simulink model "CarLike_Robot"  (R2024b)
settings: Solver=FixedStepAuto  StartTime=0.0  StopTime=T_max  FixedStep=Ts  RelTol=1e-3
StopFcn:
  | %plot_trajectory(out.x.Data(:,1), out.y.Data(:,1), 'x [m]', 'y [m]', fullfile('C:\Users\paolo\OneDrive - MSFT\Documenti\Personali\Scuola\università\magistrale\2° ANNO\Secondo Semestre\FSR\Project\Software\Images\Paper\Chapter_4_simulation\RSC\simulink', 'current_trajectory.pdf'));
  | %plot_trajectory(out.x_d.Data(1,:), out.y_d.Data(1,:), '$x_d$ [m]', '$y_d$ [m]', fullfile('C:\Users\paolo\OneDrive - MSFT\Documenti\Personali\Scuola\università\magistrale\2° ANNO\Secondo Semestre\FSR\Project\Software\Images\Paper\Chapter_4_simulation\RSC\simulink', 'desidered_trajectory.pdf'));
  | %plot_velocity(out.v.Time, out.omega.Time, out.v.Data(:,1), out.omega.Data(:,1), 'time [s]', 'v [m/s]', '$\omega$ [rad/s]', fullfile('C:\Users\paolo\OneDrive - MSFT\Documenti\Personali\Scuola\università\magistrale\2° ANNO\Secondo Semestre\FSR\Project\Software\Images\Paper\Chapter_4_simulation\RSC\simulink', 'velocity.pdf'));
  | %plot_error(out.x.Time, out.x_d.Data(1,:), out.x.Data(:,1), 'time [s]', '$e_x$ [m]', fullfile('C:\Users\paolo\OneDrive - MSFT\Documenti\Personali\Scuola\università\magistrale\2° ANNO\Secondo Semestre\FSR\Project\Software\Images\Paper\Chapter_4_simulation\RSC\simulink', 'error_x.pdf'));
  | %plot_error(out.y.Time, out.y_d.Data(1,:), out.y.Data(:,1), 'time [s]', '$e_y$ [m]', fullfile('C:\Users\paolo\OneDrive - MSFT\Documenti\Personali\Scuola\università\magistrale\2° ANNO\Secondo Semestre\FSR\Project\Software\Images\Paper\Chapter_4_simulation\RSC\simulink', 'error_y.pdf'));
  | %plot_error(out.theta.Time, out.theta_d.Data(1,:), out.theta.Data(:,1), 'time [s]', '$e_{\theta}$ [rad]', fullfile('C:\Users\paolo\OneDrive - MSFT\Documenti\Personali\Scuola\università\magistrale\2° ANNO\Secondo Semestre\FSR\Project\Software\Images\Paper\Chapter_4_simulation\RSC\simulink', 'error_theta.pdf'));
  | %plot_error(out.phi.Time, out.phi_d.Data(1,:), out.phi.Data(:,1), 'time [s]', '$e_{\phi}$ [rad]', fullfile('C:\Users\paolo\OneDrive - MSFT\Documenti\Personali\Scuola\università\magistrale\2° ANNO\Secondo Semestre\FSR\Project\Software\Images\Paper\Chapter_4_simulation\RSC\simulink', 'error_phi.pdf'));
values from neighbouring files (symbols this model uses):
  Delta = 0.2    [main.m]
  l = 0.6    [main.m]
  landmarks = zeros(num_landmarks, 2)    [main.m]
  localization = choice - 1    [main.m]
  omega_max_ref = max(abs(omega))    [main.m]
  P0 = eye(4) * 0.1    [main.m]
  q0 = [xd0; yd0; thetad0; phid0]    [main.m]
  Q_ekf = diag([0.01, 0.01])    [main.m]
  R_ekf = diag([0.05, 0.02])    [main.m]
  Ts = 0.01    [main.m]
  v_max_ref = max(abs(v))    [main.m]
  y_1d_goal = xd_end + l*cos(thetad_end) + Delta*cos(thetad_end + phid_end)    [main.m]
  y_2d_goal = yd_end + l*sin(thetad_end) + Delta*sin(thetad_end + phid_end)    [main.m]
libraries: robotmobilelib x1
settings Model: LastModifiedBy=lowan
settings SolverCC: EnableFixedStepZeroCrossing=on
settings ModelReferenceCC: EnableRefExpFcnMdlSchedulingChecks=on
settings RTWCC: GPUComputeCapability=3.5

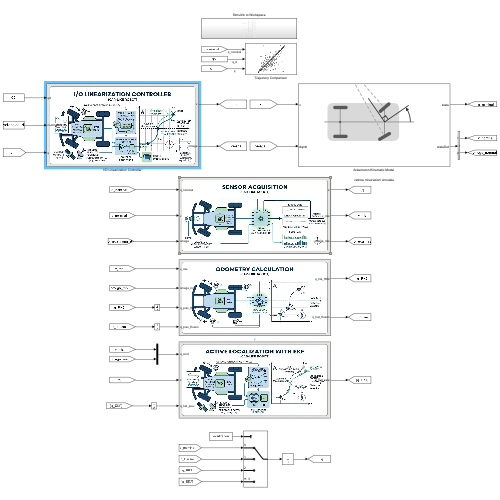
[thumbnail: Simulink's stored preview of the top-level diagram]
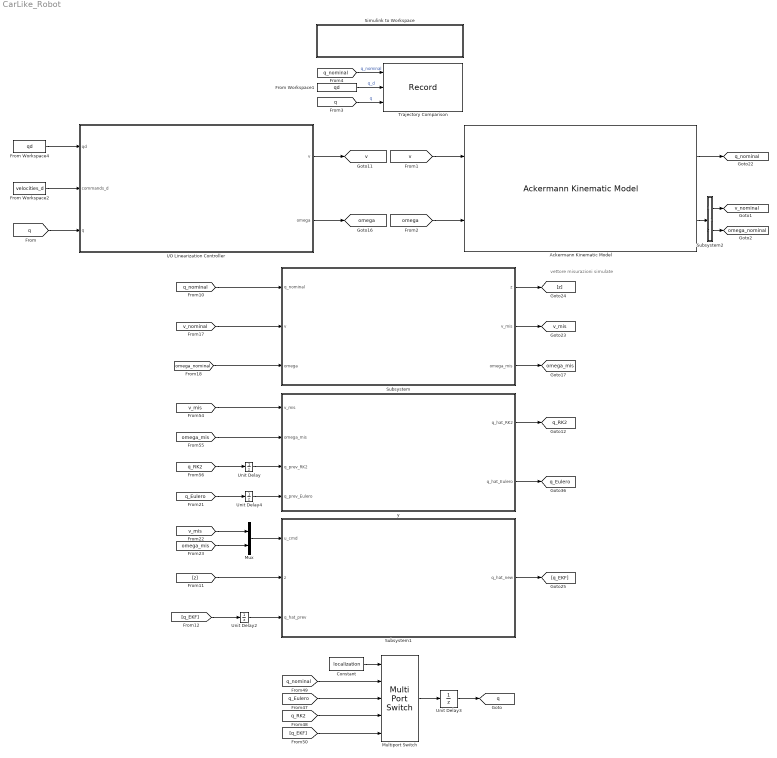
== system CarLike_Robot ==
  note: vettore misurazioni simulate
  "Ackermann Kinematic Model " : robotmobilelib/Ackermann Kinematic Model  WheelBase=0.6  VehicleSpeedRange=[-3 3]  MaxSteeringAngle=pi/4  InitialState=q0  SimulateUsing=Interpreted execution
  Constant : Constant  Value=localization
  From Workspace1 : FromWorkspace  VariableName=qd  SampleTime=Ts  OutputAfterFinalValue=Holding final value
  From Workspace2 : FromWorkspace  VariableName=velocities_d  SampleTime=Ts  OutputAfterFinalValue=Holding final value
  From Workspace4 : FromWorkspace  VariableName=qd  SampleTime=Ts  OutputAfterFinalValue=Holding final value
  I/O Linearization Controller : Subsystem
      mask Display: image('IO_Linearization_Controller.png');
  Multiport Switch : MultiPortSwitch  DataPortOrder=Zero-based contiguous  Inputs=4  zeroidx=on  SaturateOnIntegerOverflow=off  InputSameDT=off
  Mux : Mux  Inputs=2
  Simulink to Workspace : Subsystem
  Subsystem : Subsystem
      mask Display: image('Sensors.png');
  Subsystem1 : Subsystem
      mask Display: image('Active_Localization_EKF.png');
  Subsystem2 : Subsystem
  Trajectory Comparison : Record  FileSettingsInternal="{\"entries\":[{\"content\":{\"excelSettings\":{\"content\":{},\"type\":\"Streamout.ExcelSettings\"}},\"type\":\"Streamout.FileSettingStorage\",\"uuid\":\"\"}],\"packageUris\":[\"http:\\/\\/schema.mathworks.com\\/mf0\\/streamout_blocks\\/R2020a\"],\"version\":\"1.0\"}"  Layout=[1 1]  SignalsInternal="{\"entries\":[{\"content\":{\"signals\":[{\"content\":{\"blockPath\":[],\"dimensions\":[4],\"domain\":\"\",\"hasChildren\":true,\"lineColor\":\"#ff6929\",\"lineWidth\":2,\"port\":1,\"sid\":[\"\"],\"signalID\":1,\"signalName\":\"q_nominal\"},\"type\":\"RecordBlkView.Signal\",\"uuid\":\"\"},{\"content\":{\"blockPath\":[],\"channel\":[1],\"dimensions\":[4],\"domain\":\"\",\"lineColor\":\"#139fff\",\"lineWidth\":2,\"parentID\":1,\"plots\":[ 1 ],\"port\":1,\"sid\":[\"\"],\"signalID\":2,\"signalName\":\"q_nominal\"},\"type\":\"RecordBlkView.Signal\",\"uuid\":\"\"},{\"content\":{\"blockPath\":[],\"dimensions\":[4],\"domain\":\"\",\"hasChildren\":true,\"lineColor\":\"#64d413\",\"lineWidth\":2,\"port\":2,\"sid\":[\"\"],\"signalID\":3,\"signalName\":\"q_d\"},\"type\":\"RecordBlkView.Signal\",\"uuid\":\"\"},{\"content\":{\"blockPath\":[],\"channel\":[1],\"dimensions\":[4],\"domain\":\"\",\"lineColor\":\"#b746ff\",\"lineWidth\":2,\"parentID\":3,\"plots\":[ 1 ],\"port\":2,\"sid\":[\"\"],\"signalID\":4,\"signalName\":\"q_d\"},\"type\":\"RecordBlkView.Signal\",\"uuid\":\"\"},{\"content\":{\"blockPath\":[],\"dimensions\":[4,1],\"domain\":\"\",\"hasChildren\":true,\"lineColor\":\"#fe330a\",\"lineWidth\":2,\"port\":3,\"sid\":[\"\"],\"signalID\":5,\"signalName\":\"q\"},\"type\":\"RecordBlkView.Signal\",\"uuid\":\"\"},{\"content\":{\"blockPath\":[],\"channel\":[1,1],\"dimensions\":[4,1],\"domain\":\"\",\"lineColor\":\"#4dbeee\",\"lineWidth\":2,\"parentID\":5,\"plots\":[ 1 ],\"port\":3,\"sid\":[\"\"],\"signalID\":6,\"signalName\":\"q\"},\"type\":\"RecordBlkView.Signal\",\"uuid\":\"\"},{\"content\":{\"blockPath\":[],\"channel\":[2],\"dimensions\":[4],\"domain\":\"\",\"lineColor\":\"#a2142f\",\"lineWidth\":2,\"parentID\":1,\"plots\":[ 1 ],\"port\":1,\"sid\":[\"\"],\"signalID\":7,\"signalName\":\"q_nominal\"},\"type\":\"RecordBlkView.Signal\",\"uuid\":\"\"},{\"content\":{\"blockPath\":[],\"channel\":[3],\"dimensions\":[4],\"domain\":\"\",\"lineColor\":\"#139fff\",\"lineWidth\":2,\"parentID\":1,\"port\":1,\"sid\":[\"\"],\"signalID\":8,\"signalName\":\"q_nominal\"},\"type\":\"RecordBlkView.Signal\",\"uuid\":\"\"},{\"content\":{\"blockPath\":[],\"channel\":[4],\"dimensions\":[4],\"domain\":\"\",\"lineColor\":\"#ff6929\",\"lineWidth\":2,\"parentID\":1,\"port\":1,\"sid\":[\"\"],\"signalID\":9,\"signalName\":\"q_nominal\"},\"type\":\"RecordBlkView.Signal\",\"uuid\":\"\"},{\"content\":{\"blockPath\":[],\"channel\":[2],\"dimensions\":[4],\"domain\":\"\",\"lineColor\":\"#b746ff\",\"lineWidth\":2,\"parentID\":3,\"plots\":[ 1 ],\"port\":2,\"sid\":[\"\"],\"signalID\":10,\"signalName\":\"q_d\"},\"type\":\"RecordBlkView.Signal\",\"uuid\":\"\"},{\"content\":{\"blockPath\":[],\"channel\":[3],\"dimensions\":[4],\"domain\":\"\",\"lineColor\":\"#64d413\",\"lineWidth\":2,\"parentID\":3,\"port\":2,\"sid\":[\"\"],\"signalID\":11,\"signalName\":\"q_d\"},\"type\":\"RecordBlkView.Signal\",\"uuid\":\"\"},{\"content\":{\"blockPath\":[],\"channel\":[4],\"dimensions\":[4],\"domain\":\"\",\"lineColor\":\"#ff13a6\",\"lineWidth\":2,\"parentID\":3,\"port\":2,\"sid\":[\"\"],\"signalID\":12,\"signalName\":\"q_d\"},\"type\":\"RecordBlkView.Signal\",\"uuid\":\"\"},{\"content\":{\"blockPath\":[],\"channel\":[2,1],\"dimensions\":[4,1],\"domain\":\"\",\"lineColor\":\"#ff6929\",\"lineWidth\":2,\"parentID\":5,\"plots\":[ 1 ],\"port\":3,\"sid\":[\"\"],\"signalID\":13,\"signalName\":\"q\"},\"type\":\"RecordBlkView.Signal\",\"uuid\":\"\"},{\"content\":{\"blockPath\":[],\"channel\":[3,1],\"dimensions\":[4,1],\"domain\":\"\",\"lineColor\":\"#b746ff\",\"lineWidth\":2,\"parentID\":5,\"port\":3,\"sid\":[\"\"],\"signalID\":14,\"signalName\":\"q\"},\"type\":\"RecordBlkView.Signal\",\"uuid\":\"\"},{\"content\":{\"blockPath\":[],\"channel\":[4,1],\"dimensions\":[4,1],\"domain\":\"\",\"lineColor\":\"#64d413\",\"lineWidth\":2,\"parentID\":5,\"port\":3,\"sid\":[\"\"],\"signalID\":15,\"signalName\":\"q\"},\"type\":\"RecordBlkView.Signal\",\"uuid\":\"\"}]},\"type\":\"RecordBlkView.InputSignals\",\"uuid\":\"\"}],\"packageUris\":[\"http:\\/\\/schema.mathworks.com\\/mf0\\/streamout_blocks\\/R2020a\"],\"version\":\"1.0\"}"  VisualizationBindings="{\"xyplotplugin\":{\"info\":[{\"series\":[{\"bindingParametersList\":[{\"parameter\":\"X-Axis\",\"signalID\":2,\"signalName\":\"q_nominal(1)\"},{\"parameter\":\"Y-Axis\",\"signalID\":7,\"signalName\":\"q_nominal(2)\"}],\"seriesID\":0},{\"bindingParametersList\":[{\"parameter\":\"X-Axis\",\"signalID\":6,\"signalName\":\"q(1,1)\"},{\"parameter\":\"Y-Axis\",\"signalID\":13,\"signalName\":\"q(2,1)\"}],\"seriesID\":1},{\"bindingParametersList\":[{\"parameter\":\"X-Axis\",\"signalID\":4,\"signalName\":\"q_d(1)\"},{\"parameter\":\"Y-Axis\",\"signalID\":10,\"signalName\":\"q_d(2)\"}],\"seriesID\":2}],\"subplotID\":1}]}}"  CompatibilityTag=XY
  Unit Delay{,2..4} (4 alike) : UnitDelay  InitialCondition=q0  SampleTime=Ts  HasFrameUpgradeWarning=on
  y : Subsystem
      mask Display: image('Odometry.png');
  tag scope: omega=global, omega_mis=global, omega_nominal=global, q=global, q_Eulero=global, q_RK2=global, q_nominal=global, v=global, v_mis=global, v_nominal=global
  wires:
  "Ackermann Kinematic Model "/1 -> [q_nominal]
  [q_RK2] -> Unit Delay/1
  [q_EKF] -> Unit Delay2/1
  [v_mis] -> Mux/1
  [omega_mis] -> Mux/2
  [q_Eulero] -> Unit Delay4/1
  [v_mis] -> y/1(v_mis)
  [omega_mis] -> y/2(omega_mis)
  Unit Delay/1 -> y/3(q_prev_RK2)
  Unit Delay4/1 -> y/4(q_prev_Eulero)
  y/1(q_hat_RK2) -> [q_RK2]
  y/2(q_hat_Eulero) -> [q_Eulero]
  [q_nominal] -> Subsystem/1(q_nominal)
  [v_nominal] -> Subsystem/2(v)
  [omega_nominal] -> Subsystem/3(omega)
  Subsystem/1(z) -> [z]
  Subsystem/2(v_mis) -> [v_mis]
  Subsystem/3(omega_mis) -> [omega_mis]
  [omega] -> "Ackermann Kinematic Model "/2
  [q_nominal] -> Multiport Switch/2
  [q_Eulero] -> Multiport Switch/3
  [q_RK2] -> Multiport Switch/4
  [q_EKF] -> Multiport Switch/5
  Constant/1 -> Multiport Switch/1
  Multiport Switch/1 -> Unit Delay3/1
  Unit Delay3/1 -> [q]
  From Workspace4/1 -> I/O Linearization Controller/1(qd)
  [q] -> I/O Linearization Controller/3(q)
  I/O Linearization Controller/1(v) -> [v]
  I/O Linearization Controller/2(omega) -> [omega]
  Mux/1 -> Subsystem1/1(u_cmd)
  [z] -> Subsystem1/2(z)
  Unit Delay2/1 -> Subsystem1/3(q_hat_prev)
  Subsystem1/1(q_hat_new) -> [q_EKF]
  [v] -> "Ackermann Kinematic Model "/1
  From Workspace1/1 -> Trajectory Comparison/2  "q_d"
  [q_nominal] -> Trajectory Comparison/1  "q_nominal"
  From Workspace2/1 -> I/O Linearization Controller/2(commands_d)
  [q] -> Trajectory Comparison/3  "q"
  "Ackermann Kinematic Model "/2 -> Subsystem2/1(In1)
  Subsystem2/1(Out1) -> [v_nominal]
  Subsystem2/2(Out2) -> [omega_nominal]

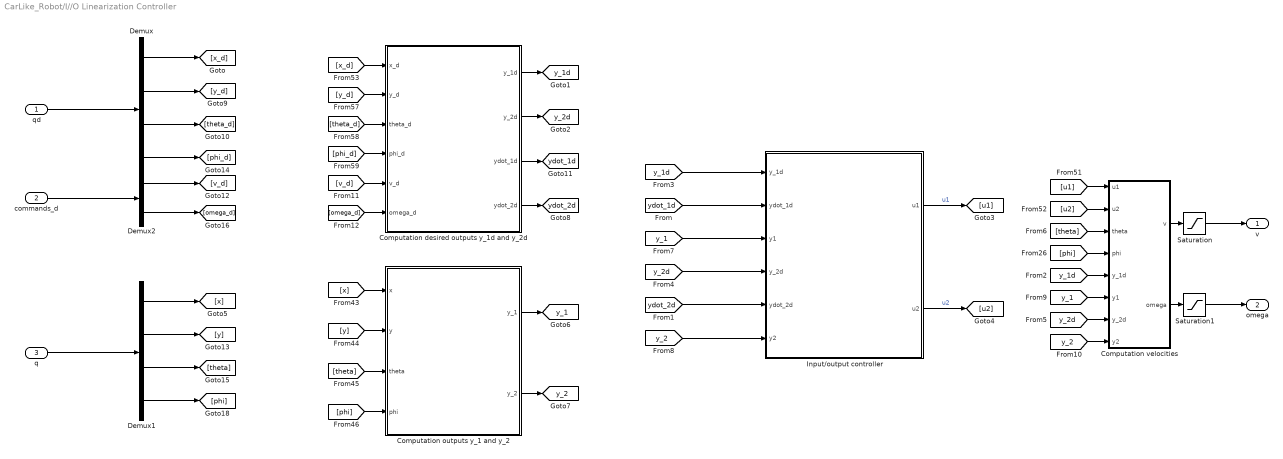
== system CarLike_Robot/I//O Linearization Controller ==
  qd : Inport
  commands_d : Inport  Port=2
  q : Inport  Port=3
  Computation desired outputs y_1d and y_2d : MATLAB Function  TreatAsAtomicUnit=on
  Computation outputs y_1 and y_2 : MATLAB Function  TreatAsAtomicUnit=on
  Computation velocities : MATLAB Function  TreatAsAtomicUnit=on
  Demux : Demux
  Demux1 : Demux
  Demux2 : Demux  Outputs=2
  Input/output controller : MATLAB Function  TreatAsAtomicUnit=on
  Saturation : Saturate  UpperLimit=v_max_ref  LowerLimit=-v_max_ref
  Saturation1 : Saturate  UpperLimit=omega_max_ref  LowerLimit=-omega_max_ref
  v : Outport
  omega : Outport  Port=2
  tag scope: y_1=global, y_1d=global, y_2=global, y_2d=global, ydot_1d=global, ydot_2d=global
  wires:
  [y_2] -> Input/output controller/6(y2)
  qd/1 -> Demux/1
  Computation desired outputs y_1d and y_2d/1(y_1d) -> [y_1d]
  [u1] -> Computation velocities/1(u1)
  [y_2d] -> Input/output controller/4(y_2d)
  [theta] -> Computation outputs y_1 and y_2/3(theta)
  Demux1/2 -> [y]
  [phi] -> Computation velocities/4(phi)
  [theta] -> Computation velocities/3(theta)
  [x] -> Computation outputs y_1 and y_2/1(x)
  Demux1/4 -> [phi]
  [y_1d] -> Input/output controller/1(y_1d)
  Computation outputs y_1 and y_2/2(y_2) -> [y_2]
  [phi] -> Computation outputs y_1 and y_2/4(phi)
  [y] -> Computation outputs y_1 and y_2/2(y)
  Computation outputs y_1 and y_2/1(y_1) -> [y_1]
  [phi_d] -> Computation desired outputs y_1d and y_2d/4(phi_d)
  Demux/4 -> [phi_d]
  Demux/2 -> [y_d]
  [y_1] -> Input/output controller/3(y1)
  Input/output controller/2(u2) -> [u2]  "u2"
  [u2] -> Computation velocities/2(u2)
  Computation desired outputs y_1d and y_2d/2(y_2d) -> [y_2d]
  Input/output controller/1(u1) -> [u1]  "u1"
  [x_d] -> Computation desired outputs y_1d and y_2d/1(x_d)
  Demux/1 -> [x_d]
  Demux1/3 -> [theta]
  [theta_d] -> Computation desired outputs y_1d and y_2d/3(theta_d)
  q/1 -> Demux1/1
  Demux/3 -> [theta_d]
  [y_d] -> Computation desired outputs y_1d and y_2d/2(y_d)
  Demux1/1 -> [x]
  Computation velocities/1(v) -> Saturation/1
  Computation velocities/2(omega) -> Saturation1/1
  Saturation/1 -> v/1
  Saturation1/1 -> omega/1
  commands_d/1 -> Demux2/1
  Computation desired outputs y_1d and y_2d/4(ydot_2d) -> [ydot_2d]
  Computation desired outputs y_1d and y_2d/3(ydot_1d) -> [ydot_1d]
  [ydot_1d] -> Input/output controller/2(ydot_1d)
  [ydot_2d] -> Input/output controller/5(ydot_2d)
  [y_2] -> Computation velocities/8(y2)
  [y_1] -> Computation velocities/6(y1)
  [y_2d] -> Computation velocities/7(y_2d)
  [y_1d] -> Computation velocities/5(y_1d)
  Demux2/1 -> [v_d]
  Demux2/2 -> [omega_d]
  [v_d] -> Computation desired outputs y_1d and y_2d/5(v_d)
  [omega_d] -> Computation desired outputs y_1d and y_2d/6(omega_d)

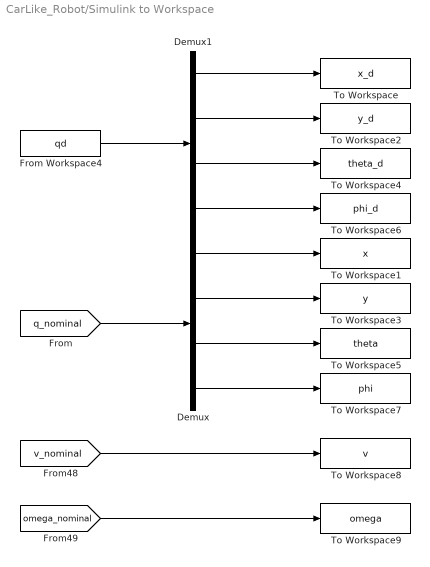
== system CarLike_Robot/Simulink to Workspace ==
  Demux : Demux
  Demux1 : Demux
  From Workspace4 : FromWorkspace  VariableName=qd  SampleTime=Ts  OutputAfterFinalValue=Holding final value
  To Workspace : ToWorkspace  VariableName=x_d  SaveFormat=Timeseries  SampleTime=-1
  To Workspace1 : ToWorkspace  VariableName=x  SaveFormat=Timeseries  SampleTime=-1
  To Workspace2 : ToWorkspace  VariableName=y_d  SaveFormat=Timeseries  SampleTime=-1
  To Workspace3 : ToWorkspace  VariableName=y  SaveFormat=Timeseries  SampleTime=-1
  To Workspace4 : ToWorkspace  VariableName=theta_d  SaveFormat=Timeseries  SampleTime=-1
  To Workspace5 : ToWorkspace  VariableName=theta  SaveFormat=Timeseries  SampleTime=-1
  To Workspace6 : ToWorkspace  VariableName=phi_d  SaveFormat=Timeseries  SampleTime=-1
  To Workspace7 : ToWorkspace  VariableName=phi  SaveFormat=Timeseries  SampleTime=-1
  To Workspace8 : ToWorkspace  VariableName=v  SaveFormat=Timeseries  SampleTime=-1
  To Workspace9 : ToWorkspace  VariableName=omega  SaveFormat=Timeseries  SampleTime=-1
  wires:
  [v_nominal] -> To Workspace8/1
  [omega_nominal] -> To Workspace9/1
  [q_nominal] -> Demux/1
  Demux/1 -> To Workspace1/1
  Demux/2 -> To Workspace3/1
  Demux/3 -> To Workspace5/1
  Demux/4 -> To Workspace7/1
  Demux1/1 -> To Workspace/1
  Demux1/2 -> To Workspace2/1
  Demux1/3 -> To Workspace4/1
  Demux1/4 -> To Workspace6/1
  From Workspace4/1 -> Demux1/1

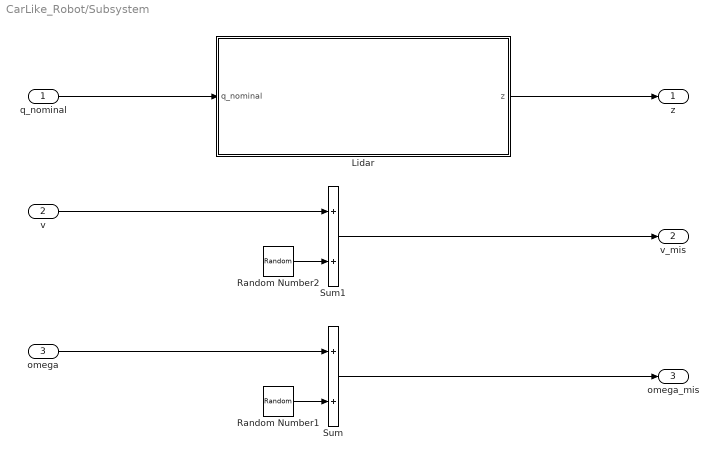
== system CarLike_Robot/Subsystem ==
  q_nominal : Inport
  v : Inport  Port=2
  omega : Inport  Port=3
  Lidar : MATLAB Function  TreatAsAtomicUnit=on
  Random Number1 : RandomNumber  Variance=1e-6  Seed=10  SampleTime=Ts
  Random Number2 : RandomNumber  Variance=1e-6  SampleTime=Ts
  Sum : Sum
  Sum1 : Sum
  z : Outport
  v_mis : Outport  Port=2
  omega_mis : Outport  Port=3
  wires:
  omega/1 -> Sum/1
  Sum1/1 -> v_mis/1
  v/1 -> Sum1/1
  Lidar/1(z) -> z/1
  q_nominal/1 -> Lidar/1(q_nominal)
  Sum/1 -> omega_mis/1
  Random Number2/1 -> Sum1/2
  Random Number1/1 -> Sum/2

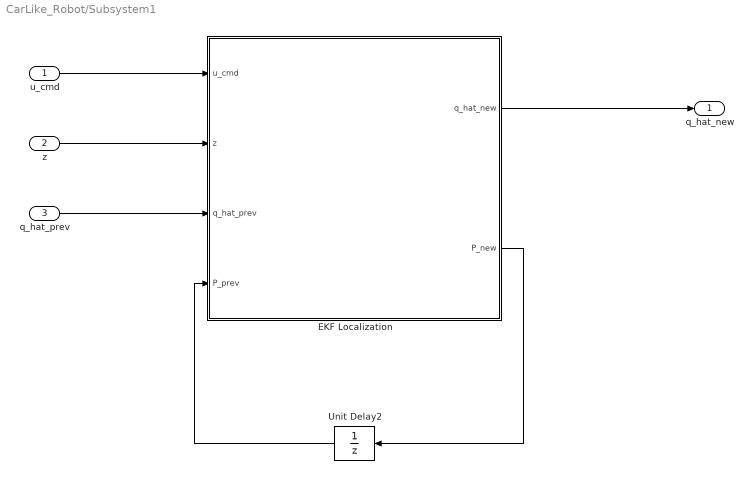
== system CarLike_Robot/Subsystem1 ==
  u_cmd : Inport
  z : Inport  Port=2
  q_hat_prev : Inport  Port=3
  EKF Localization : MATLAB Function  TreatAsAtomicUnit=on
  Unit Delay2 : UnitDelay  InitialCondition=P0  SampleTime=Ts  HasFrameUpgradeWarning=on
  q_hat_new : Outport
  wires:
  q_hat_prev/1 -> EKF Localization/3(q_hat_prev)
  z/1 -> EKF Localization/2(z)
  Unit Delay2/1 -> EKF Localization/4(P_prev)
  EKF Localization/2(P_new) -> Unit Delay2/1
  u_cmd/1 -> EKF Localization/1(u_cmd)
  EKF Localization/1(q_hat_new) -> q_hat_new/1

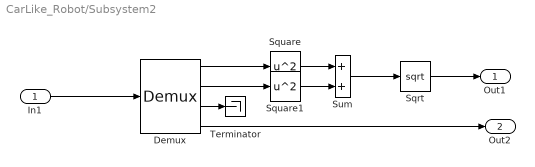
== system CarLike_Robot/Subsystem2 ==
  In1 : Inport
  Demux : Demux
      settings: DisplayOption=none
  Sqrt : Sqrt
  Square : Math  Operator=square
  Square1 : Math  Operator=square
  Sum : Sum
  Terminator : Terminator
  Out1 : Outport
  Out2 : Outport  Port=2
  wires:
  Sum/1 -> Sqrt/1
  Square1/1 -> Sum/2
  Demux/3 -> Terminator/1
  Demux/4 -> Out2/1
  Demux/1 -> Square/1
  Demux/2 -> Square1/1
  Square/1 -> Sum/1
  In1/1 -> Demux/1
  Sqrt/1 -> Out1/1

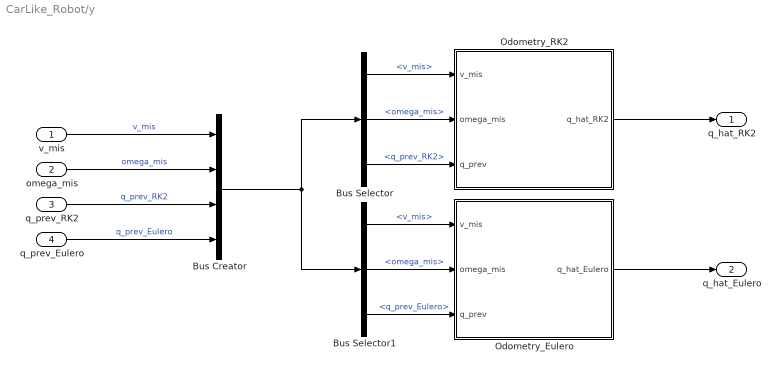
== system CarLike_Robot/y ==
  v_mis : Inport
  omega_mis : Inport  Port=2
  q_prev_RK2 : Inport  Port=3
  q_prev_Eulero : Inport  Port=4
  Bus Creator : BusCreator  Inputs=4
  Bus Selector : BusSelector  OutputSignals=v_mis,omega_mis,q_prev_RK2
  Bus Selector1 : BusSelector  OutputSignals=v_mis,omega_mis,q_prev_Eulero
  Odometry_Eulero : MATLAB Function  TreatAsAtomicUnit=on
  Odometry_RK2 : MATLAB Function  TreatAsAtomicUnit=on
  q_hat_RK2 : Outport
  q_hat_Eulero : Outport  Port=2
  wires:
  Bus Creator/1 -> Bus Selector1/1, Bus Selector/1
  Bus Selector1/1 -> Odometry_Eulero/1(v_mis)  "<v_mis>"
  Bus Selector1/2 -> Odometry_Eulero/2(omega_mis)  "<omega_mis>"
  Bus Selector/3 -> Odometry_RK2/3(q_prev)  "<q_prev_RK2>"
  Bus Selector/1 -> Odometry_RK2/1(v_mis)  "<v_mis>"
  Bus Selector/2 -> Odometry_RK2/2(omega_mis)  "<omega_mis>"
  Odometry_RK2/1(q_hat_RK2) -> q_hat_RK2/1
  Bus Selector1/3 -> Odometry_Eulero/3(q_prev)  "<q_prev_Eulero>"
  omega_mis/1 -> Bus Creator/2  "omega_mis"
  q_prev_RK2/1 -> Bus Creator/3  "q_prev_RK2"
  v_mis/1 -> Bus Creator/1  "v_mis"
  q_prev_Eulero/1 -> Bus Creator/4  "q_prev_Eulero"
  Odometry_Eulero/1(q_hat_Eulero) -> q_hat_Eulero/1

== matlab function CarLike_Robot/Subsystem1/EKF Localization ==
  data: u_cmd input; z input; q_hat_prev input; P_prev input; q_hat_new output; P_new output; Ts parameter; l parameter; landmarks parameter; Q_ekf parameter; R_ekf parameter
function [q_hat_new, P_new] = fcn(u_cmd, z, q_hat_prev, P_prev, Ts, l, landmarks, Q_ekf, R_ekf)
    % EKF per Car-Like Robot
    
    v = u_cmd(1);
    omega = u_cmd(2);
    
    x = q_hat_prev(1);
    y = q_hat_prev(2);
    theta = q_hat_prev(3);
    phi = q_hat_prev(4);
    
    %% --- PREDICTION STEP (Odometria RK2) ---
    % 1. Predizione dello stato (Runge-Kutta 2)
    phi_m = phi + 0.5 * omega * Ts;
    th_m = theta + 0.5 * (v / l) * tan(phi) * Ts;
    
    q_pred = zeros(4,1);
    q_pred(1) = x + v * Ts * cos(th_m);
    q_pred(2) = y + v * Ts * sin(th_m);
    q_pred(3) = theta + (v / l) * tan(phi_m) * Ts;
    q_pred(4) = phi + omega * Ts;
    
    % 2. Jacobiana del modello di moto rispetto allo stato (F)
    % (Approssimazione di Eulero per la covarianza)
    F = eye(4);
    F(1,3) = -v * sin(theta) * Ts;
    F(2,3) = v * cos(theta) * Ts;
    F(3,4) = (v/l) * (1 / (cos(phi)^2)) * Ts;
    
    % 3. Jacobiana del modello rispetto agli ingressi (W)
    W = zeros(4,2);
    W(1,1) = cos(theta) * Ts;
    W(2,1) = sin(theta) * Ts;
    W(3,1) = (1/l) * tan(phi) * Ts;
    W(4,2) = Ts;
    
    % 4. Propagazione Covarianza
    P_pred = F * P_prev * F' + W * Q_ekf * W';
    
    %% --- UPDATE STEP (LIDAR) ---
    num_landmarks = size(landmarks, 1);
    q_hat_new = q_pred;
    P_new = P_pred;
    
    % Aggiornamento sequenziale per ogni landmark
    for i = 1:num_landmarks
        Lx = landmarks(i, 1);
        Ly = landmarks(i, 2);
        
        dx = Lx - q_hat_new(1);
        dy = Ly - q_hat_new(2);
        rho2 = dx^2 + dy^2;
        rho = sqrt(rho2);
        
        if rho > 0.1 % Evita singolarità
            % Misurazione attesa
            z_hat = [rho; atan2(dy, dx) - q_hat_new(3)];
            z_hat(2) = atan2(sin(z_hat(2)), cos(z_hat(2)));
            
            % Jacobiana del modello di misura (H)
            H = zeros(2, 4);
            H(1,1) = -dx / rho;
            H(1,2) = -dy / rho;
            H(2,1) = dy / rho2;
            H(2,2) = -dx / rho2;
            H(2,3) = -1;
            
            % Innovazione
            z_meas = z(2*i-1 : 2*i);
            y_res = z_meas - z_hat;
            y_res(2) = atan2(sin(y_res(2)), cos(y_res(2)));
            
            % Kalman Gain
            S = H * P_new * H' + R_ekf;
            K = P_new * H' / S;
            
            % Update Stato e Covarianza
            q_hat_new = q_hat_new + K * y_res;
            P_new = (eye(4) - K * H) * P_new;
        end
    end
end

== matlab function CarLike_Robot/y/Odometry_Eulero ==
  data: v_mis input; q_hat_Eulero output; omega_mis input; q_prev input; l parameter; Ts parameter
function q_hat_Eulero = fcn(v_mis, omega_mis, q_prev, l, Ts)
    % Estrazione stati al passo k
    x_k = q_prev(1);
    y_k = q_prev(2);
    th_k = q_prev(3);
    phi_k = q_prev(4);
    
    % Integrazione con metodo di Eulero in avanti
    x_next = x_k + v_mis * Ts * cos(th_k);
    y_next = y_k + v_mis * Ts * sin(th_k);
    th_next = th_k + (v_mis / l) * tan(phi_k) * Ts;
    phi_next = phi_k + omega_mis * Ts;
    
    % Aggiornamento vettore di stato
    q_hat_Eulero = [x_next; y_next; th_next; phi_next];
end

== matlab function CarLike_Robot/I//O Linearization Controller/Computation desired outputs y_1d and y_2d ==
  data: x_d input; y_1d output; y_d input; theta_d input; phi_d input; v_d input; omega_d input; y_2d output; l parameter; Delta parameter; ydot_1d output; ydot_2d output
function [y_1d, y_2d, ydot_1d, ydot_2d] = fcn(x_d, y_d, theta_d, phi_d, v_d, omega_d, l, Delta)
    
    % 1. Calcolo delle posizioni desiderate (come prima)
    y_1d = x_d + l*cos(theta_d) + Delta*cos(theta_d+phi_d);
    y_2d = y_d + l*sin(theta_d) + Delta*sin(theta_d+phi_d);
    
    % 2. Calcolo Analitico Esatto delle Derivate (Niente più spike!)
    % Usiamo la matrice di trasformazione cinematica T(theta, phi) del Car-Like
    
    T11 = cos(theta_d) - tan(phi_d)*sin(theta_d) - (Delta/l)*tan(phi_d)*sin(theta_d+phi_d);
    T12 = -Delta * sin(theta_d+phi_d);
    
    T21 = sin(theta_d) + tan(phi_d)*cos(theta_d) + (Delta/l)*tan(phi_d)*cos(theta_d+phi_d);
    T22 =  Delta * cos(theta_d+phi_d);
    
    % Le derivate sono l'esatta proiezione delle velocità di riferimento
    ydot_1d = T11 * v_d + T12 * omega_d;
    ydot_2d = T21 * v_d + T22 * omega_d;

end

== matlab function CarLike_Robot/I//O Linearization Controller/Computation velocities ==
  data: u1 input; v output; omega output; u2 input; theta input; phi input; l parameter; Delta parameter; y_1d input; y1 input; y_2d input; y2 input; y_1d_goal parameter; y_2d_goal parameter
function [v, omega] = fcn(u1, u2, theta, phi, l, Delta, y_1d, y1, y_2d, y2, y_1d_goal, y_2d_goal)
    % --- Trasformazione cinematica inversa (invariata) ---
    T = [cos(theta)-tan(phi)*(sin(theta)+(Delta*sin(theta+phi))/l) -Delta*sin(theta+phi);
         sin(theta)+tan(phi)*(cos(theta)+(Delta*cos(theta+phi))/l) +Delta*cos(theta+phi)];
    Tinv = inv(T);
    v_raw = Tinv(1,:)*[u1; u2];
    omega_raw = Tinv(2,:)*[u1; u2];

    % --- Logica di "arrivo": smorzamento dolce SOLO vicino al goal finale ---
    % Distanza del riferimento corrente (y_1d,y_2d) dal punto finale della traiettoria.
    % Quando questa distanza e' grande, siamo ancora "in viaggio": damp=1, nessun
    % effetto. Solo quando il riferimento stesso e' arrivato al goal (perche' la
    % traiettoria e' finita, q_goal_finale raggiunto) iniziamo a smorzare in base
    % all'errore di tracking residuo, cosi' il rumore di misura vicino alla
    % singolarita' di T non viene piu' amplificato in comandi v,omega enormi.
    dist_from_goal = sqrt((y_1d - y_1d_goal)^2 + (y_2d - y_2d_goal)^2);

    d_hi = 0.15;   % m: sopra questa distanza dal goal, siamo ancora in viaggio
    d_lo = 0.05;   % m: sotto questa distanza, il riferimento e' "arrivato"

    if dist_from_goal >= d_hi
        near_goal = 0;   % comportamento normale, niente smorzamento
    elseif dist_from_goal <= d_lo
        near_goal = 1;   % riferimento fermo sul goal
    else
        frac = (dist_from_goal - d_lo) / (d_hi - d_lo);
        near_goal = 0.5 * (1 + cos(pi * frac));  % 1 a d_lo, 0 a d_hi, C1
    end

    % Solo quando near_goal=1 applichiamo lo smorzamento sull'errore residuo di
    % tracking (che a quel punto e' solo rumore di misura, non un transitorio
    % legittimo di inseguimento traiettoria).
    err = sqrt((y_1d - y1)^2 + (y_2d - y2)^2);
    e_hi = 0.10;
    e_lo = 0.02;
    if err >= e_hi
        damp_err = 1;
    elseif err <= e_lo
        damp_err = 0;
    else
        frac_e = (err - e_lo) / (e_hi - e_lo);
        damp_err = 0.5 * (1 - cos(pi * frac_e));
    end

    % Fattore di smorzamento complessivo: 1 (nessun effetto) lontano dal goal,
    % oppure vicino al goal ma con errore ancora significativo (transitorio di
    % arrivo); scende verso damp_err SOLO quando near_goal=1 e l'errore e' piccolo.
    damp = 1 - near_goal * (1 - damp_err);

    v = damp * v_raw;
    omega = damp * omega_raw;
end

== matlab function CarLike_Robot/I//O Linearization Controller/Input//output controller ==
  data: y_1d input; u1 output; ydot_1d input; y1 input; y_2d input; ydot_2d input; y2 input; u2 output
function [u1, u2] = fcn(y_1d, ydot_1d, y1, y_2d, ydot_2d, y2)

k1 = 15; 
k2 = 15; 

u1 = ydot_1d+k1*(y_1d-y1);
u2 = ydot_2d+k2*(y_2d-y2);

end

== matlab function CarLike_Robot/I//O Linearization Controller/Computation outputs y_1 and y_2 ==
  data: x input; y_1 output; y input; theta input; phi input; y_2 output; l parameter; Delta parameter
function [y_1, y_2]  = fcn(x, y, theta, phi, l, Delta)

y_1 = x+l*cos(theta)+Delta*cos(theta+phi);
y_2 = y+l*sin(theta)+Delta*sin(theta+phi);

end

== matlab function CarLike_Robot/Subsystem/Lidar ==
  settings: updateMethod=DISCRETE
  data: q_nominal input; z output; R_ekf parameter; landmarks parameter
function z = fcn(q_nominal, R_ekf, landmarks)
    % q_real = [x; y; theta; phi] reale dal modello Ackermann
    % z = Vettore colonna delle misurazioni [r1; alpha1; r2; alpha2; ...]
    
    % --- MASCHERA DI AVVIO ---
    persistent startup_ticks
    if isempty(startup_ticks)
        startup_ticks = 5; % Per i primi 5 passi (0.05s) non mettiamo rumore
    end
    
    noise_mult = 1;
    if startup_ticks > 0
        noise_mult = 0; % Azzera il rumore
        startup_ticks = startup_ticks - 1;
    end
    % -------------------------

    num_landmarks = size(landmarks, 1);
    z = zeros(num_landmarks * 2, 1);
    
    x = q_nominal(1);
    y = q_nominal(2);
    theta = q_nominal(3);
    
    for i = 1:num_landmarks
        Lx = landmarks(i, 1);
        Ly = landmarks(i, 2);
        
        % Distanza vera
        r_true = sqrt((Lx - x)^2 + (Ly - y)^2);
        % Angolo vero relativo al robot
        alpha_true = atan2(Ly - y, Lx - x) - theta;
        
        % Normalizzazione angolo
        alpha_true = atan2(sin(alpha_true), cos(alpha_true));
        
        % Aggiunta rumore gaussiano MOLTIPLICATO per la maschera
        r_noisy = r_true + noise_mult * sqrt(R_ekf(1,1)) * randn();
        alpha_noisy = alpha_true + noise_mult * sqrt(R_ekf(2,2)) * randn();
        
        z(2*i - 1) = r_noisy;
        z(2*i) = alpha_noisy;
    end
end

== matlab function CarLike_Robot/y/Odometry_RK2 ==
  data: v_mis input; q_hat_RK2 output; omega_mis input; q_prev input; l parameter; Ts parameter
function q_hat_RK2 = fcn(v_mis, omega_mis, q_prev, l, Ts)
    % Estrazione stati al passo k
    x_k = q_prev(1);
    y_k = q_prev(2);
    th_k = q_prev(3);
    phi_k = q_prev(4);
    
    % STEP 1: Calcolo degli stati al punto medio (midpoint)
    phi_m = phi_k + 0.5 * omega_mis * Ts;
    th_m = th_k + 0.5 * (v_mis / l) * tan(phi_k) * Ts;
    
    % STEP 2: Integrazione RK2 (usando gli angoli del punto medio)
    x_next = x_k + v_mis * Ts * cos(th_m);
    y_next = y_k + v_mis * Ts * sin(th_m);
    th_next = th_k + (v_mis / l) * tan(phi_m) * Ts;
    phi_next = phi_k + omega_mis * Ts;
    
    % Aggiornamento vettore di stato
    q_hat_RK2 = [x_next; y_next; th_next; phi_next];
end
